simulink model "test_serial_com_PIX"  (R2018a)
settings: Solver=FixedStepAuto  StartTime=0.0  StopTime=10.0  RelTol=1e-3
undefined symbols (not defined in the file): RGBLED_COLOR_ENUM, RGBLED_MODE_ENUM
libraries: etargetslib x2, pixhawk_slib_ADC_serial x2, pixhawk_slib_sensors_actuators x1
settings Model: Creator=hiepp  LastModifiedBy=hiepp
settings OptimizationCC: DefaultParameterBehavior=Inlined  EnhancedBackFolding=on  PassReuseOutputArgsAs=Individual arguments  MaxStackSize=64  OptimizeBlockOrder=speed  DifferentSizesBufferReuse=on  OptimizationCustomize=off
settings DebuggingCC: ParameterTunabilityLossMsg=error
settings HardwareCC: ProdBitPerPointer=32  ProdBitPerSizeT=32  ProdBitPerPtrDiffT=32  ProdLargestAtomicInteger=Long  ProdLargestAtomicFloat=Double  ProdWordSize=32  ProdHWDeviceType=ARM Compatible->ARM Cortex
settings SFSimCC: MATLABDynamicMemAlloc=off
settings RTWCC: SystemTargetFile=ert.tlc  HardwareBoard=Pixhawk PX4  TLCOptions="-aInlineSetEventsForThisBaseRateFcn=TLC_FALSE -aSuppressMultiTaskScheduler=TLC_FALSE  -aRateBasedStepFcn=0"  TemplateMakefile=ert_default_tmf  GenerateReport=on  Toolchain=Pixhawk Toolchain  IncludeHyperlinkInReport=on  LaunchReport=on  GenerateTraceInfo=on  GenerateTraceReport=on  GenerateTraceReportSl=on  GenerateTraceReportSf=on  GenerateTraceReportEml=on
settings CodeAppCC: ForceParamTrailComments=on  IgnoreCustomStorageClasses=off  OperatorAnnotations=on  SimulinkDataObjDesc=on  SFDataObjDesc=on  InsertBlockDesc=on
settings ERTTargetCC: ERTCustomFileTemplate=PX4_codertarget_file_process.tlc

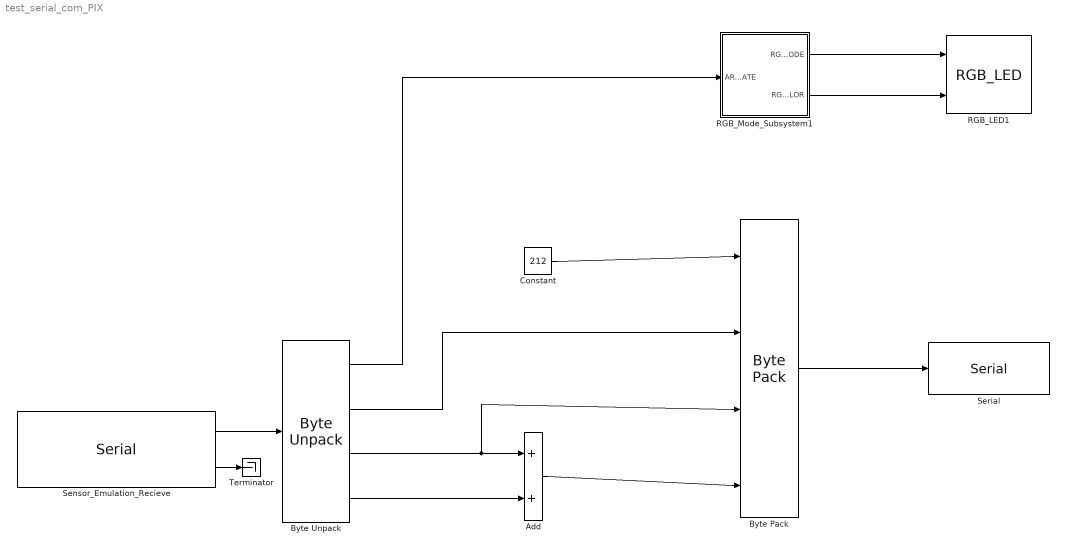
== system test_serial_com_PIX ==
  Add : Sum
  Byte Pack : etargetslib/Byte Pack  datatypes={'single','single','single','single'}  byteAlign=1
  Byte Unpack : etargetslib/Byte Unpack  dimensions={[1],[1],[1],[1],}  datatypes={'single','single','single','single'}  byteAlign=1
  Constant : Constant  Value=212  OutDataTypeStr=single
  RGB_LED1 : pixhawk_slib_sensors_actuators/RGB_LED
      settings: SourceProductName=Pixhawk Target Blocks
  RGB_Mode_Subsystem1 : Subsystem
  Sensor_Emulation_Recieve : pixhawk_slib_ADC_serial/Serial  DeviceName=/dev/ttyS5  ReadOrWrite=Reading  BaudRateStr=115200  block=off  WriteStatus=on  Terminator=off  Header=off  NumBytesRead=16  TerminatorChar=\n  HeaderData=[ uint8( hex2dec( 'DE' ) ), uint8( hex2dec( 'AD' ) ), uint8( hex2dec( 'C0' ) ), uint8( hex2dec( 'DE' ) ) ]  SimulateUsing=Code generation
      settings: SourceProductName=Pixhawk Target Blocks
  Serial : pixhawk_slib_ADC_serial/Serial  DeviceName=/dev/ttyS5  ReadOrWrite=Writing  BaudRateStr=115200  block=off  WriteStatus=on  Terminator=off  Header=off  NumBytesRead=4  TerminatorChar=\n  HeaderData=[ uint8( hex2dec( 'DE' ) ), uint8( hex2dec( 'AD' ) ), uint8( hex2dec( 'C0' ) ), uint8( hex2dec( 'DE' ) ) ]  SimulateUsing=Code generation
      settings: SourceProductName=Pixhawk Target Blocks
  Terminator : Terminator
  wires:
  Sensor_Emulation_Recieve/1 -> Byte Unpack/1
  Sensor_Emulation_Recieve/2 -> Terminator/1
  Byte Unpack/3 -> Byte Pack/3, Add/1
  Byte Unpack/4 -> Add/2
  Add/1 -> Byte Pack/4
  RGB_Mode_Subsystem1/2(RGB_COLOR) -> RGB_LED1/2
  Byte Unpack/1 -> RGB_Mode_Subsystem1/1(ARM_STATE)
  Constant/1 -> Byte Pack/1
  Byte Unpack/2 -> Byte Pack/2
  RGB_Mode_Subsystem1/1(RGB_MODE) -> RGB_LED1/1
  Byte Pack/1 -> Serial/1

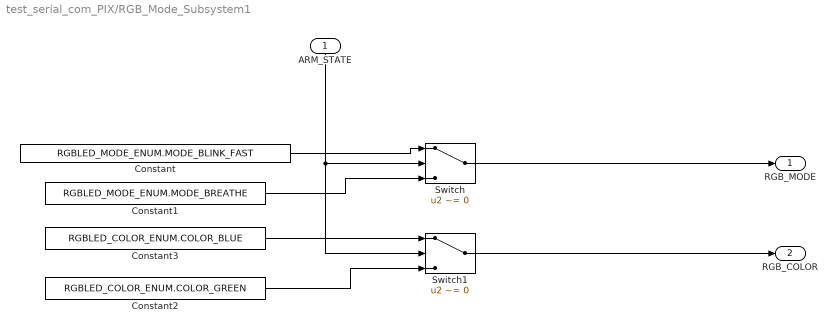
== system test_serial_com_PIX/RGB_Mode_Subsystem1 ==
  ARM_STATE : Inport
  Constant : Constant  Value=RGBLED_MODE_ENUM.MODE_BLINK_FAST  OutDataTypeStr=Enum: RGBLED_MODE_ENUM
  Constant1 : Constant  Value=RGBLED_MODE_ENUM.MODE_BREATHE  OutDataTypeStr=Enum: RGBLED_MODE_ENUM
  Constant2 : Constant  Value=RGBLED_COLOR_ENUM.COLOR_GREEN  OutDataTypeStr=Enum: RGBLED_COLOR_ENUM
  Constant3 : Constant  Value=RGBLED_COLOR_ENUM.COLOR_BLUE  OutDataTypeStr=Enum: RGBLED_COLOR_ENUM
  Switch : Switch  Criteria=u2 ~= 0  Threshold=1500
  Switch1 : Switch  Criteria=u2 ~= 0  Threshold=1500
  RGB_MODE : Outport
  RGB_COLOR : Outport  Port=2
  wires:
  Switch1/1 -> RGB_COLOR/1
  Constant2/1 -> Switch1/3
  Constant3/1 -> Switch1/1
  Switch/1 -> RGB_MODE/1
  Constant1/1 -> Switch/3
  Constant/1 -> Switch/1
  ARM_STATE/1 -> Switch/2, Switch1/2
